simulink model "reaktor_liniowy"  (R2016a)
settings: Solver=VariableStepAuto  StartTime=0.0  StopTime=10.0  RelTol=1e-3
values from neighbouring files (symbols this model uses):
  LAMBDA = 10 ^ -5    (= 1e-05)    [Unit_3.m]    (also in reactor_pocz.m; unit_1.m; unit_4.m)
  N = 99.3    [Unit_3.m]    (also in unit_1.m = 100.3; unit_4.m = 100.8)
undefined symbols (not defined in the file or in its folder): p_1, p_2, p_3
settings Model: Creator=Michal Chruscinski  LastModifiedBy=Michal Chruscinski

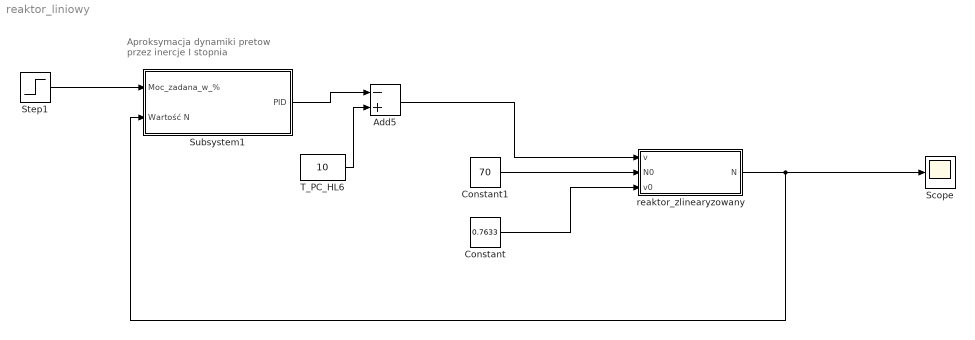
== system reaktor_liniowy ==
  note: Aproksymacja dynamiki
      | pretow przez inercje I stopnia
  Add5 : Sum  Inputs=-+
  Constant : Constant  Value=0.7633
  Constant1 : Constant  Value=70
  Scope : Scope
  Step1 : Step  Time=5  Before=60  After=70  SampleTime=0
  Subsystem1 : Subsystem
  T_PC_HL6 : Constant  Value=10
  reaktor_zlinearyzowany : Subsystem
  wires:
  Add5/1 -> reaktor_zlinearyzowany/1(v)
  Constant/1 -> reaktor_zlinearyzowany/3(v0)
  Constant1/1 -> reaktor_zlinearyzowany/2(N0)
  Step1/1 -> Subsystem1/1(Moc_zadana_w_%)
  reaktor_zlinearyzowany/1(N) -> Subsystem1/2(Wartość N), Scope/1
  Subsystem1/1("PID ") -> Add5/1
  T_PC_HL6/1 -> Add5/2

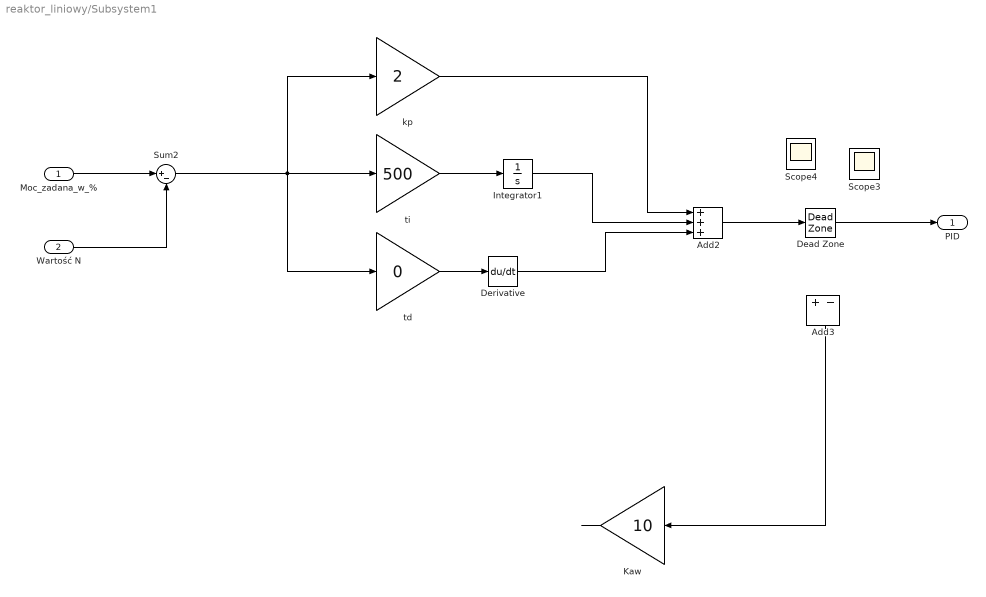
== system reaktor_liniowy/Subsystem1 ==
  Moc_zadana_w_% : Inport
  Wartość N : Inport  Port=2
  " kp " : Gain  Gain=2
  Add2 : Sum  Inputs=+++
  Add3 : Sum  Inputs=+-
  Dead Zone : DeadZone  LowerValue=-10  UpperValue=0  SaturateOnIntegerOverflow=on
  Derivative : Derivative
  Integrator1 : Integrator
  "Kaw " : Gain  Gain=10
  Scope3 : Scope
  Scope4 : Scope
  Sum2 : Sum  Inputs=|+-
  "td " : Gain  Gain=0
  ti : Gain  Gain=500
  "PID " : Outport
  wires:
  "td "/1 -> Derivative/1
  Add3/1 -> "Kaw "/1
  " kp "/1 -> Add2/1
  ti/1 -> Integrator1/1
  Integrator1/1 -> Add2/2
  Derivative/1 -> Add2/3
  Sum2/1 -> "td "/1, " kp "/1, ti/1
  Add2/1 -> Dead Zone/1
  "Kaw "/1 -> ?
  ? -> Scope4/1
  ? -> Scope3/1
  Dead Zone/1 -> "PID "/1
  Moc_zadana_w_%/1 -> Sum2/1
  Wartość N/1 -> Sum2/2

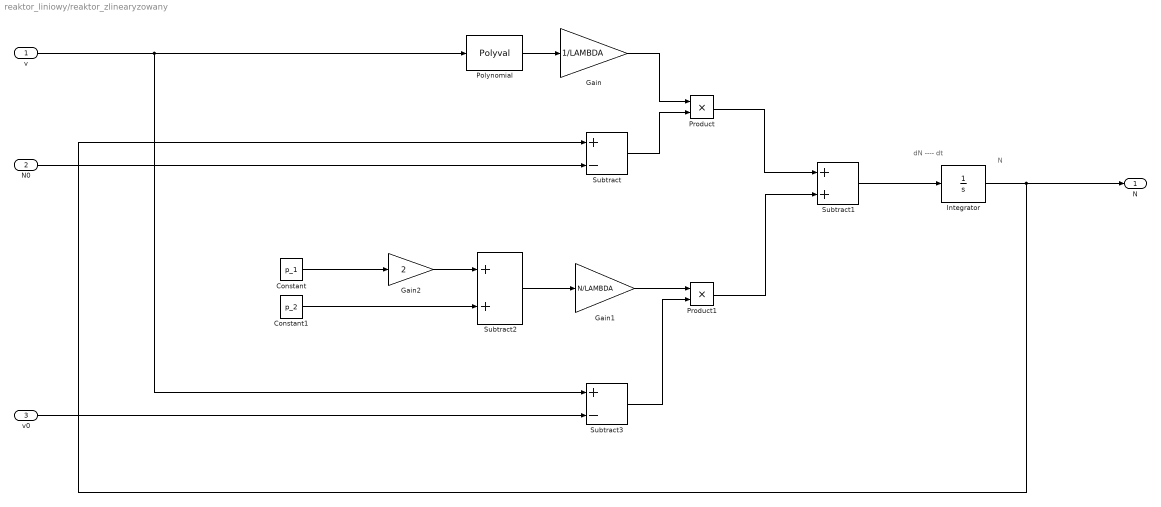
== system reaktor_liniowy/reaktor_zlinearyzowany ==
  note: N
  note: dN
      | ----
      | dt
  v : Inport
  N0 : Inport  Port=2
  v0 : Inport  Port=3
  Constant : Constant  Value=p_1
  Constant1 : Constant  Value=p_2
  Gain : Gain  Gain=1/LAMBDA
  Gain1 : Gain  Gain=N/LAMBDA
  Gain2 : Gain  Gain=2
  Integrator : Integrator
  Polynomial : Polyval  Coefs=[ p_1, p_2, p_3 ]
  Product : Product
  Product1 : Product
  Subtract : Sum  Inputs=+-
  Subtract1 : Sum
  Subtract2 : Sum
  Subtract3 : Sum  Inputs=+-
  N : Outport
  wires:
  Polynomial/1 -> Gain/1
  N0/1 -> Subtract/2
  v/1 -> Subtract3/1, Polynomial/1
  Subtract/1 -> Product/2
  Gain/1 -> Product/1
  Product/1 -> Subtract1/1
  Subtract2/1 -> Gain1/1
  Gain2/1 -> Subtract2/1
  Constant/1 -> Gain2/1
  Constant1/1 -> Subtract2/2
  Gain1/1 -> Product1/1
  Subtract3/1 -> Product1/2
  Product1/1 -> Subtract1/2
  v0/1 -> Subtract3/2
  Subtract1/1 -> Integrator/1
  Integrator/1 -> N/1, Subtract/1
